simulink model "FLCU_Gauging_Test_Harness_Permittivity"  (R2019b)
settings: Solver=FixedStepAuto  StartTime=0.0  StopTime=10  FixedStep=0.02  RelTol=1e-3
settings Model: DataDictionary=FLCU_Gauging.sldd  Creator=aymanouchker  LastModifiedBy=aymanouchker
settings DataIOCC: SignalLoggingName=BusData
settings OptimizationCC: DefaultParameterBehavior=Inlined  UseDivisionForNetSlopeComputation=on  GainParamInheritBuiltInType=on  UseFloatMulNetSlope=on  DefaultUnderspecifiedDataType=single  UseSpecifiedMinMax=on  InlineInvariantSignals=on  EnhancedBackFolding=on  CachingGlobalReferences=on  PassReuseOutputArgsAs=Individual arguments  StateBitsets=on  DataBitsets=on  ZeroExternalMemoryAtStartup=off  ZeroInternalMemoryAtStartup=off  NoFixptDivByZeroProtection=on  EfficientFloat2IntCast=on  LifeSpan=inf  OptimizeBlockOrder=speed  DifferentSizesBufferReuse=on  EfficientTunableParamExpr=on
settings DebuggingCC: SignalInfNanChecking=warning  IntegerOverflowMsg=error  ParameterTunabilityLossMsg=error  UniqueDataStoreMsg=error  AssertControl=DisableAll  StrictBusMsg=ErrorOnBusTreatedAsVector  SFUndirectedBroadcastEventsDiag=error
settings HardwareCC: ProdBitPerInt=16  ProdBitPerPointer=16  ProdBitPerSizeT=16  ProdBitPerPtrDiffT=16  ProdLargestAtomicFloat=None  ProdWordSize=16  ProdLongLongMode=on  ProdHWDeviceType=STMicroelectronics->ST10/Super10
settings SFSimCC: CompileTimeRecursionLimit=0  EnableRuntimeRecursion=off  MATLABDynamicMemAlloc=off
settings RTWCC: SystemTargetFile=ert.tlc  TemplateMakefile=ert_default_tmf  GenerateReport=on  BuildConfiguration=Faster Runs  IncludeHyperlinkInReport=on  LaunchReport=on  GenerateTraceInfo=on  GenerateTraceReport=on  GenerateTraceReportSl=on  GenerateTraceReportSf=on  GenerateTraceReportEml=on
settings CodeAppCC: ForceParamTrailComments=on  IgnoreCustomStorageClasses=off  IgnoreTestpoints=on  OperatorAnnotations=on  SimulinkDataObjDesc=on  SFDataObjDesc=on  MATLABFcnDesc=on  InsertBlockDesc=on  StateflowObjectComments=on  MATLABSourceComments=on  EnableCustomComments=on  ReqsInCode=on
settings ERTTargetCC: TargetLangStandard=C99 (ISO)  UtilityFuncGeneration=Shared location  GenerateSampleERTMain=on  CombineSignalStateStructs=on  SuppressErrorStatus=on  SupportAbsoluteTime=off  MultiInstanceERTCode=on  CodeInterfacePackaging=Reusable function  SupportNonFinite=off  ParenthesesLevel=Maximum  CastingMode=Standards  GenerateSharedConstants=off  InlinedParameterPlacement=NonHierarchical  ERTCustomFileTemplate=example_file_process.tlc  PreserveExpressionOrder=on  PreserveIfCondition=on  EnableSignedLeftShifts=off  EnableSignedRightShifts=off

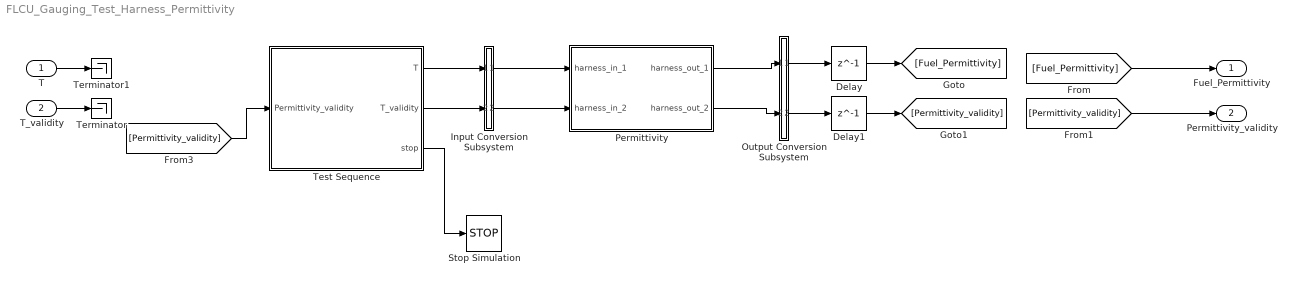
== system FLCU_Gauging_Test_Harness_Permittivity ==
  T : Inport  OutDataTypeStr=double  PortDimensions=[1]  SampleTime=[-1, 0]
  T_validity : Inport  Port=2  OutMin=0  OutMax=1  OutDataTypeStr=boolean  PortDimensions=[1]  SampleTime=[-1, 0]
  Delay : Delay  DelayLength=1
  Delay1 : Delay  DelayLength=1
  Input Conversion Subsystem : Subsystem  Tag=__SLT_ICS__  Description=|
      | Signal spec.
      | and routing
      settings: AttributesFormatString=%<Description>
  Output Conversion Subsystem : Subsystem  Tag=__SLT_OCS__  Description=|
      | Signal spec.
      | and routing
      settings: AttributesFormatString=%<Description>
  Permittivity : Subsystem  Tag=__SL_testing_harness_stub_
  Stop Simulation : Stop
  Terminator : Terminator
  Terminator1 : Terminator
  Test Sequence : Test Sequence  TreatAsAtomicUnit=on
  Fuel_Permittivity : Outport
  Permittivity_validity : Outport  Port=2
  wires:
  Input Conversion Subsystem/1(Outport_1) -> Permittivity/1(harness_in_1)
  Input Conversion Subsystem/2(Outport_2) -> Permittivity/2(harness_in_2)
  Permittivity/1(harness_out_1) -> Output Conversion Subsystem/1(Inport_1)
  Permittivity/2(harness_out_2) -> Output Conversion Subsystem/2(Inport_2)
  T_validity/1 -> Terminator/1
  T/1 -> Terminator1/1
  Output Conversion Subsystem/2(Outport_2) -> Delay1/1
  Output Conversion Subsystem/1(Outport_1) -> Delay/1
  Delay/1 -> [Fuel_Permittivity]
  Delay1/1 -> [Permittivity_validity]
  [Fuel_Permittivity] -> Fuel_Permittivity/1
  [Permittivity_validity] -> Permittivity_validity/1
  [Permittivity_validity] -> Test Sequence/1(Permittivity_validity)
  Test Sequence/1(T) -> Input Conversion Subsystem/1(Inport_1)
  Test Sequence/2(T_validity) -> Input Conversion Subsystem/2(Inport_2)
  Test Sequence/3(stop) -> Stop Simulation/1

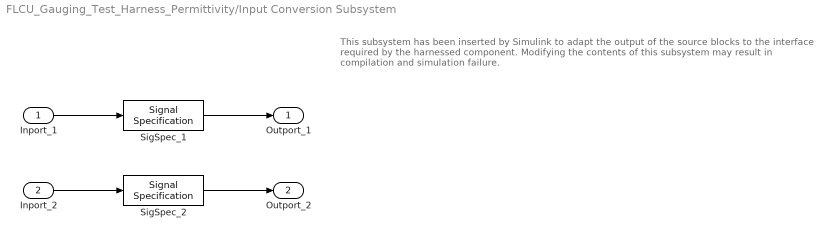
== system FLCU_Gauging_Test_Harness_Permittivity/Input Conversion Subsystem ==
  note: This subsystem has been inserted by Simulink to adapt the output of the source blocks to the interface required by the harnessed component.
      |  Modifying the contents of this subsystem may result in compilation and simulation failure.
  Inport_1 : Inport
  Inport_2 : Inport  Port=2
  SigSpec_1 : SignalSpecification  OutDataTypeStr=double  Unit=°C  Dimensions=[1]  SampleTime=[-1, 0]
  SigSpec_2 : SignalSpecification  OutDataTypeStr=boolean  Dimensions=[1]  SampleTime=[-1, 0]
  Outport_1 : Outport
  Outport_2 : Outport  Port=2
  wires:
  SigSpec_1/1 -> Outport_1/1
  Inport_1/1 -> SigSpec_1/1
  SigSpec_2/1 -> Outport_2/1
  Inport_2/1 -> SigSpec_2/1

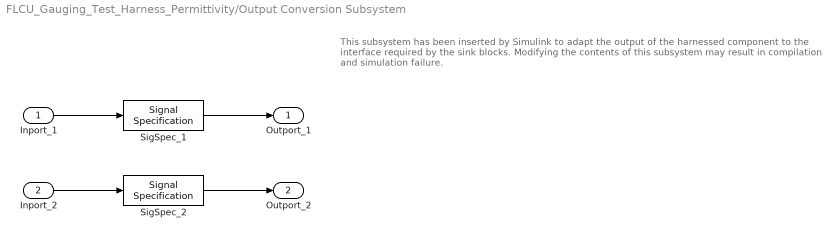
== system FLCU_Gauging_Test_Harness_Permittivity/Output Conversion Subsystem ==
  note: This subsystem has been inserted by Simulink to adapt the output of the harnessed component to the interface required by the sink blocks.
      |  Modifying the contents of this subsystem may result in compilation and simulation failure.
  Inport_1 : Inport
  Inport_2 : Inport  Port=2
  SigSpec_1 : SignalSpecification  OutDataTypeStr=double  Dimensions=[1]
  SigSpec_2 : SignalSpecification  OutDataTypeStr=boolean  Dimensions=[1]
  Outport_1 : Outport
  Outport_2 : Outport  Port=2
  wires:
  Inport_1/1 -> SigSpec_1/1
  SigSpec_1/1 -> Outport_1/1
  Inport_2/1 -> SigSpec_2/1
  SigSpec_2/1 -> Outport_2/1

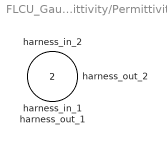
== system FLCU_Gauging_Test_Harness_Permittivity/Permittivity ==
  harness_in_1 : Inport
  harness_in_2 : Inport  Port=2
  harness_out_1 : Outport
  harness_out_2 : Outport  Port=2

== stateflow chart FLCU_Gauging_Test_Harness_Permittivity/Test Sequence ==
  settings: stateMachineType=SIMPLIFIED_MACHINE
  state Initialization
    T=0;
    T_validity=true;
    stop=false;
    count=0;
  state step_1
    T=1;
    T_validity=true;
  state step_2
    verify(Permittivity_validity==true);
  state step_3
    T=34;
    T_validity=true;
  state step_4
    count=count+1;
    verify(Permittivity_validity==false);
  state step_5
    T=14;
    T_validity=false;
  state step_6
    stop=true;
  (default) -> Initialization
  Initialization -> step_1
  step_1 -> step_2
  step_2 -> step_3
  step_3 -> step_4
  step_4 -> (junction 39) [order 2] : [
      | count==2
      | ]
  (junction 39) -> (junction 37)
  step_4 -> step_5 [order 1] : [
      | count==1
      | ]
  step_5 -> step_4
  (junction 37) -> step_6
  data: Permittivity_validity input; T output; T_validity output; stop output; count local
